simulink model "Exp10"  (Simulink 7.1)
settings: Solver=ode45  StartTime=0.0  StopTime=1  RelTol=1e-3
libraries: simulink x15
settings Model: Creator=George  LastModifiedBy=George

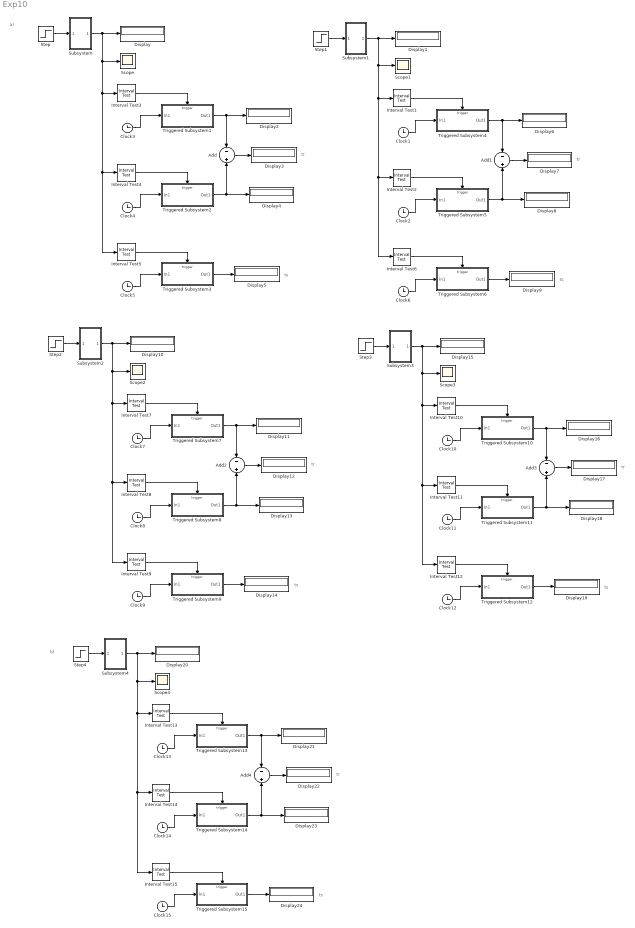
== system Exp10 ==
  note: tr
  note: ts
  note: tr
  note: ts
  note: tr
  note: ts
  note: tr
  note: ts
  note: a)
  note: tr
  note: ts
  note: b)
  Add{,1..4} (5 alike) : Sum  Inputs=-+  OutDataType=sfix(16)  OutScaling=2^-10
  Clock{1..15} (15 alike) : Clock
      settings: Decimation=10
  Display{,1..24} (25 alike) : Display
  Interval Test{1,3,7,10,13} (5 alike) : simulink/Logic and Bit Operations/Interval Test  SystemSampleTime=-1  IntervalClosedRight=on  uplimit=0.1  IntervalClosedLeft=on  lowlimit=0  LogicOutDataTypeMode=boolean
  Interval Test{2,4,8,11,14} (5 alike) : simulink/Logic and Bit Operations/Interval Test  SystemSampleTime=-1  IntervalClosedRight=on  uplimit=0.9  IntervalClosedLeft=on  lowlimit=0  LogicOutDataTypeMode=boolean
  Interval Test{5..6,9,12,15} (5 alike) : simulink/Logic and Bit Operations/Interval Test  SystemSampleTime=-1  IntervalClosedRight=on  uplimit=1.05  IntervalClosedLeft=on  lowlimit=0.95  LogicOutDataTypeMode=boolean
  Scope{,1..4} (5 alike) : Scope
      Scope2 settings: SaveName=ScopeData2
      Scope3 settings: SaveName=ScopeData3
      Scope4 settings: SaveName=ScopeData4
  Step{,1..4} (5 alike) : Step  Time=0  SampleTime=0
  Subsystem : Subsystem  mask{R1=5000, R2=5000, K=0, C1=250*10^-9, C2=250*10^-9}
  Subsystem1 : Subsystem  mask{R1=5000, R2=5000, K=0.5, C1=250*10^-9, C2=250*10^-9}
  Subsystem2 : Subsystem  mask{R1=5000, R2=5000, K=1, C1=250*10^-9, C2=250*10^-9}
  Subsystem3 : Subsystem  mask{R1=5000, R2=5000, K=2, C1=250*10^-9, C2=250*10^-9}
  Subsystem4 : Subsystem  mask{R1=5000, R2=5000, K=1, C1=250*10^-9, C2=250*10^-9}
  Triggered Subsystem1 : Subsystem  TreatAsAtomicUnit=on
  Triggered Subsystem10 : Subsystem  TreatAsAtomicUnit=on
  Triggered Subsystem11 : Subsystem  TreatAsAtomicUnit=on
  Triggered Subsystem12 : Subsystem  TreatAsAtomicUnit=on
  Triggered Subsystem13 : Subsystem  TreatAsAtomicUnit=on
  Triggered Subsystem14 : Subsystem  TreatAsAtomicUnit=on
  Triggered Subsystem15 : Subsystem  TreatAsAtomicUnit=on
  Triggered Subsystem2 : Subsystem  TreatAsAtomicUnit=on
  Triggered Subsystem3 : Subsystem  TreatAsAtomicUnit=on
  Triggered Subsystem4 : Subsystem  TreatAsAtomicUnit=on
  Triggered Subsystem5 : Subsystem  TreatAsAtomicUnit=on
  Triggered Subsystem6 : Subsystem  TreatAsAtomicUnit=on
  Triggered Subsystem7 : Subsystem  TreatAsAtomicUnit=on
  Triggered Subsystem8 : Subsystem  TreatAsAtomicUnit=on
  Triggered Subsystem9 : Subsystem  TreatAsAtomicUnit=on
  wires:
  Step/1 -> Subsystem/1(In1)
  Subsystem/1(Out1) -> Display/1, Interval Test3/1, Interval Test4/1, Interval Test5/1, Scope/1
  Clock3/1 -> Triggered Subsystem1/1(In1)
  Interval Test3/1 -> Triggered Subsystem1/Trigger
  Clock4/1 -> Triggered Subsystem2/1(In1)
  Interval Test4/1 -> Triggered Subsystem2/Trigger
  Clock5/1 -> Triggered Subsystem3/1(In1)
  Interval Test5/1 -> Triggered Subsystem3/Trigger
  Triggered Subsystem1/1(Out1) -> Add/1, Display2/1
  Triggered Subsystem2/1(Out1) -> Add/2, Display4/1
  Add/1 -> Display3/1
  Triggered Subsystem3/1(Out1) -> Display5/1
  Step1/1 -> Subsystem1/1(In1)
  Subsystem1/1(Out1) -> Display1/1, Interval Test1/1, Interval Test2/1, Interval Test6/1, Scope1/1
  Clock1/1 -> Triggered Subsystem4/1(In1)
  Interval Test1/1 -> Triggered Subsystem4/Trigger
  Clock2/1 -> Triggered Subsystem5/1(In1)
  Interval Test2/1 -> Triggered Subsystem5/Trigger
  Clock6/1 -> Triggered Subsystem6/1(In1)
  Interval Test6/1 -> Triggered Subsystem6/Trigger
  Triggered Subsystem4/1(Out1) -> Add1/1, Display6/1
  Triggered Subsystem5/1(Out1) -> Add1/2, Display8/1
  Add1/1 -> Display7/1
  Triggered Subsystem6/1(Out1) -> Display9/1
  Step2/1 -> Subsystem2/1(In1)
  Subsystem2/1(Out1) -> Display10/1, Interval Test7/1, Interval Test8/1, Interval Test9/1, Scope2/1
  Clock7/1 -> Triggered Subsystem7/1(In1)
  Interval Test7/1 -> Triggered Subsystem7/Trigger
  Clock8/1 -> Triggered Subsystem8/1(In1)
  Interval Test8/1 -> Triggered Subsystem8/Trigger
  Clock9/1 -> Triggered Subsystem9/1(In1)
  Interval Test9/1 -> Triggered Subsystem9/Trigger
  Triggered Subsystem7/1(Out1) -> Add2/1, Display11/1
  Triggered Subsystem8/1(Out1) -> Add2/2, Display13/1
  Add2/1 -> Display12/1
  Triggered Subsystem9/1(Out1) -> Display14/1
  Step3/1 -> Subsystem3/1(In1)
  Subsystem3/1(Out1) -> Display15/1, Interval Test10/1, Interval Test11/1, Interval Test12/1, Scope3/1
  Clock10/1 -> Triggered Subsystem10/1(In1)
  Interval Test10/1 -> Triggered Subsystem10/Trigger
  Clock11/1 -> Triggered Subsystem11/1(In1)
  Interval Test11/1 -> Triggered Subsystem11/Trigger
  Clock12/1 -> Triggered Subsystem12/1(In1)
  Interval Test12/1 -> Triggered Subsystem12/Trigger
  Triggered Subsystem10/1(Out1) -> Add3/1, Display16/1
  Triggered Subsystem11/1(Out1) -> Add3/2, Display18/1
  Add3/1 -> Display17/1
  Triggered Subsystem12/1(Out1) -> Display19/1
  Step4/1 -> Subsystem4/1(In1)
  Subsystem4/1(Out1) -> Display20/1, Interval Test13/1, Interval Test14/1, Interval Test15/1, Scope4/1
  Clock13/1 -> Triggered Subsystem13/1(In1)
  Interval Test13/1 -> Triggered Subsystem13/Trigger
  Clock14/1 -> Triggered Subsystem14/1(In1)
  Interval Test14/1 -> Triggered Subsystem14/Trigger
  Clock15/1 -> Triggered Subsystem15/1(In1)
  Interval Test15/1 -> Triggered Subsystem15/Trigger
  Triggered Subsystem13/1(Out1) -> Add4/1, Display21/1
  Triggered Subsystem14/1(Out1) -> Add4/2, Display23/1
  Add4/1 -> Display22/1
  Triggered Subsystem15/1(Out1) -> Display24/1

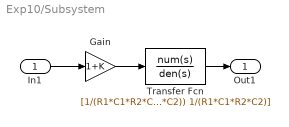
== system Exp10/Subsystem ==
  In1 : Inport
  Gain : Gain  Gain=1+K  ParameterDataType=sfix(16)  ParameterScaling=2^0  OutDataType=sfix(16)  OutScaling=2^0
  Transfer Fcn : TransferFcn  Numerator=[1/(R1*C1*R2*C2)]  Denominator=[1 (1/(R1*C1) + 1/(R2*C1) - K * 1/(R2*C2)) 1/(R1*C1*R2*C2)]
  Out1 : Outport
  wires:
  Gain/1 -> Transfer Fcn/1
  In1/1 -> Gain/1
  Transfer Fcn/1 -> Out1/1

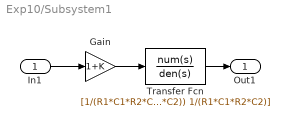
== system Exp10/Subsystem1 ==
  In1 : Inport
  Gain : Gain  Gain=1+K  ParameterDataType=sfix(16)  ParameterScaling=2^0  OutDataType=sfix(16)  OutScaling=2^0
  Transfer Fcn : TransferFcn  Numerator=[1/(R1*C1*R2*C2)]  Denominator=[1 (1/(R1*C1) + 1/(R2*C1) - K * 1/(R2*C2)) 1/(R1*C1*R2*C2)]
  Out1 : Outport
  wires:
  Gain/1 -> Transfer Fcn/1
  In1/1 -> Gain/1
  Transfer Fcn/1 -> Out1/1

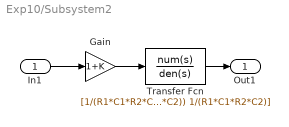
== system Exp10/Subsystem2 ==
  In1 : Inport
  Gain : Gain  Gain=1+K  ParameterDataType=sfix(16)  ParameterScaling=2^0  OutDataType=sfix(16)  OutScaling=2^0
  Transfer Fcn : TransferFcn  Numerator=[1/(R1*C1*R2*C2)]  Denominator=[1 (1/(R1*C1) + 1/(R2*C1) - K * 1/(R2*C2)) 1/(R1*C1*R2*C2)]
  Out1 : Outport
  wires:
  Gain/1 -> Transfer Fcn/1
  In1/1 -> Gain/1
  Transfer Fcn/1 -> Out1/1

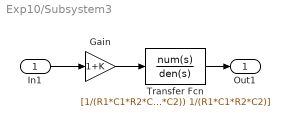
== system Exp10/Subsystem3 ==
  In1 : Inport
  Gain : Gain  Gain=1+K  ParameterDataType=sfix(16)  ParameterScaling=2^0  OutDataType=sfix(16)  OutScaling=2^0
  Transfer Fcn : TransferFcn  Numerator=[1/(R1*C1*R2*C2)]  Denominator=[1 (1/(R1*C1) + 1/(R2*C1) - K * 1/(R2*C2)) 1/(R1*C1*R2*C2)]
  Out1 : Outport
  wires:
  Gain/1 -> Transfer Fcn/1
  In1/1 -> Gain/1
  Transfer Fcn/1 -> Out1/1

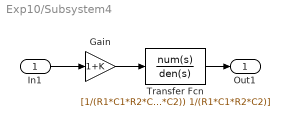
== system Exp10/Subsystem4 ==
  In1 : Inport
  Gain : Gain  Gain=1+K  ParameterDataType=sfix(16)  ParameterScaling=2^0  OutDataType=sfix(16)  OutScaling=2^0
  Transfer Fcn : TransferFcn  Numerator=[1/(R1*C1*R2*C2)]  Denominator=[1 (1/(R1*C1) + 1/(R2*C1) - K * 1/(R2*C2)) 1/(R1*C1*R2*C2)]
  Out1 : Outport
  wires:
  Gain/1 -> Transfer Fcn/1
  In1/1 -> Gain/1
  Transfer Fcn/1 -> Out1/1

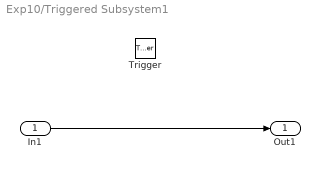
== system Exp10/Triggered Subsystem1 ==
  In1 : Inport  OutDataType=sfix(16)  OutScaling=2^0
  Trigger : TriggerPort  TriggerType=falling
  Out1 : Outport  OutDataType=sfix(16)  OutScaling=2^0
  wires:
  In1/1 -> Out1/1

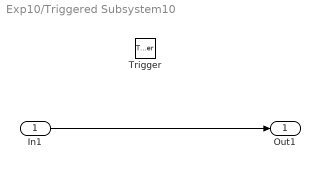
== system Exp10/Triggered Subsystem10 ==
  In1 : Inport  OutDataType=sfix(16)  OutScaling=2^0
  Trigger : TriggerPort  TriggerType=falling
  Out1 : Outport  OutDataType=sfix(16)  OutScaling=2^0
  wires:
  In1/1 -> Out1/1

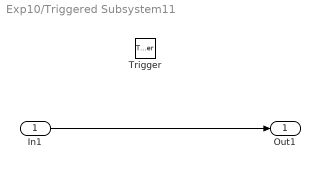
== system Exp10/Triggered Subsystem11 ==
  In1 : Inport  OutDataType=sfix(16)  OutScaling=2^0
  Trigger : TriggerPort  TriggerType=falling
  Out1 : Outport  OutDataType=sfix(16)  OutScaling=2^0
  wires:
  In1/1 -> Out1/1

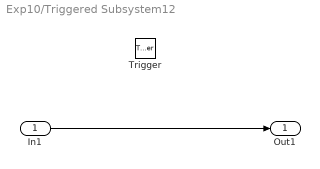
== system Exp10/Triggered Subsystem12 ==
  In1 : Inport  OutDataType=sfix(16)  OutScaling=2^0
  Trigger : TriggerPort  TriggerType=either
  Out1 : Outport  OutDataType=sfix(16)  OutScaling=2^0
  wires:
  In1/1 -> Out1/1

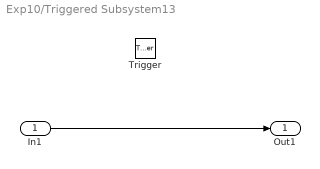
== system Exp10/Triggered Subsystem13 ==
  In1 : Inport  OutDataType=sfix(16)  OutScaling=2^0
  Trigger : TriggerPort  TriggerType=falling
  Out1 : Outport  OutDataType=sfix(16)  OutScaling=2^0
  wires:
  In1/1 -> Out1/1

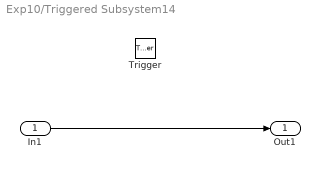
== system Exp10/Triggered Subsystem14 ==
  In1 : Inport  OutDataType=sfix(16)  OutScaling=2^0
  Trigger : TriggerPort  TriggerType=falling
  Out1 : Outport  OutDataType=sfix(16)  OutScaling=2^0
  wires:
  In1/1 -> Out1/1

== system Exp10/Triggered Subsystem15 ==
  In1 : Inport  OutDataType=sfix(16)  OutScaling=2^0
  Trigger : TriggerPort  TriggerType=either
  Out1 : Outport  OutDataType=sfix(16)  OutScaling=2^0
  wires:
  In1/1 -> Out1/1

== system Exp10/Triggered Subsystem2 ==
  In1 : Inport  OutDataType=sfix(16)  OutScaling=2^0
  Trigger : TriggerPort  TriggerType=falling
  Out1 : Outport  OutDataType=sfix(16)  OutScaling=2^0
  wires:
  In1/1 -> Out1/1

== system Exp10/Triggered Subsystem3 ==
  In1 : Inport  OutDataType=sfix(16)  OutScaling=2^0
  Trigger : TriggerPort  TriggerType=either
  Out1 : Outport  OutDataType=sfix(16)  OutScaling=2^0
  wires:
  In1/1 -> Out1/1

== system Exp10/Triggered Subsystem4 ==
  In1 : Inport  OutDataType=sfix(16)  OutScaling=2^0
  Trigger : TriggerPort  TriggerType=falling
  Out1 : Outport  OutDataType=sfix(16)  OutScaling=2^0
  wires:
  In1/1 -> Out1/1

== system Exp10/Triggered Subsystem5 ==
  In1 : Inport  OutDataType=sfix(16)  OutScaling=2^0
  Trigger : TriggerPort  TriggerType=falling
  Out1 : Outport  OutDataType=sfix(16)  OutScaling=2^0
  wires:
  In1/1 -> Out1/1

== system Exp10/Triggered Subsystem6 ==
  In1 : Inport  OutDataType=sfix(16)  OutScaling=2^0
  Trigger : TriggerPort  TriggerType=either
  Out1 : Outport  OutDataType=sfix(16)  OutScaling=2^0
  wires:
  In1/1 -> Out1/1

== system Exp10/Triggered Subsystem7 ==
  In1 : Inport  OutDataType=sfix(16)  OutScaling=2^0
  Trigger : TriggerPort  TriggerType=falling
  Out1 : Outport  OutDataType=sfix(16)  OutScaling=2^0
  wires:
  In1/1 -> Out1/1

== system Exp10/Triggered Subsystem8 ==
  In1 : Inport  OutDataType=sfix(16)  OutScaling=2^0
  Trigger : TriggerPort  TriggerType=falling
  Out1 : Outport  OutDataType=sfix(16)  OutScaling=2^0
  wires:
  In1/1 -> Out1/1

== system Exp10/Triggered Subsystem9 ==
  In1 : Inport  OutDataType=sfix(16)  OutScaling=2^0
  Trigger : TriggerPort  TriggerType=either
  Out1 : Outport  OutDataType=sfix(16)  OutScaling=2^0
  wires:
  In1/1 -> Out1/1
